simulink model "solar_powered_EV_charger"  (R2021a)
settings: Solver=VariableStepAuto  StartTime=0.0  StopTime=10.0  RelTol=1e-3
libraries: spsCurrentMeasurementLib x2, spsSeriesRLCBranchLib x2, spsVoltageMeasurementLib x2, spsDiodeLib x1, spsMosfetLib x1, spsPVArrayLib x1
settings Model: Creator=hp  LastModifiedBy=hp

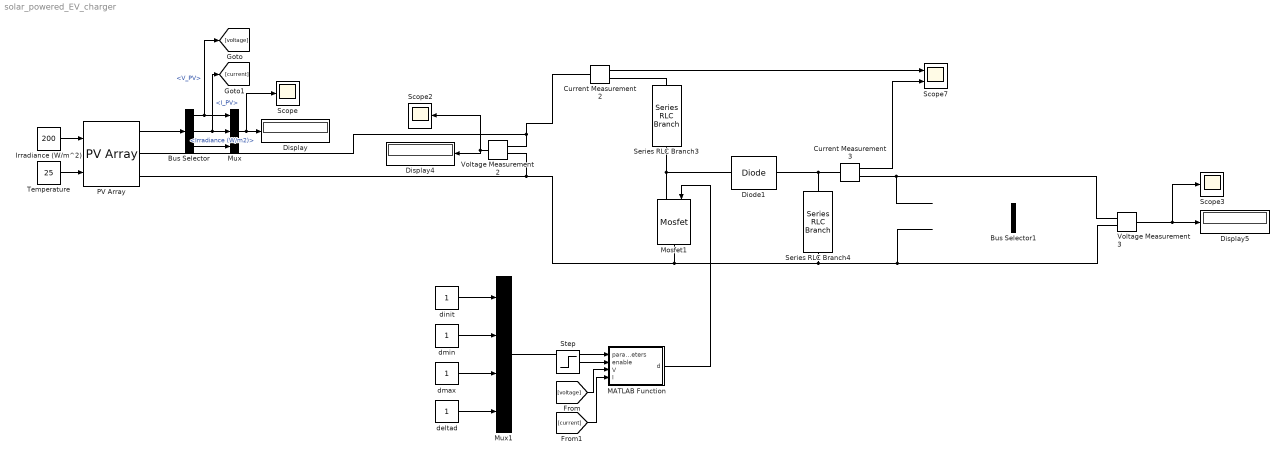
== system solar_powered_EV_charger ==
  Bus Selector : BusSelector  OutputSignals=V_PV,I_PV,Irradiance (W/m2)
  Bus Selector1 : BusSelector  OutputSignals=SOC (%),Current (A),Voltage (V)
  Current Measurement2 : spsCurrentMeasurementLib/Current Measurement  PhasorSimulation=off  OutputType=Complex  PSBequivalent=0
  Current Measurement3 : spsCurrentMeasurementLib/Current Measurement  PhasorSimulation=off  OutputType=Complex  PSBequivalent=0
  Diode1 : spsDiodeLib/Diode  Ron=0.001  Lon=0  Vf=0.8  IC=0  UseSnubber=0  Rs=500  Cs=250e-9  Measurements=off
  Display : Display
  Display4 : Display
  Display5 : Display
  Irradiance (W/m^2) : Constant  Value=200
  MATLAB Function : MATLAB Function  TreatAsAtomicUnit=on
  Mosfet1 : spsMosfetLib/Mosfet  Ron=0.1  Lon=0  Rd=0.01  Vfd=0  IC=0  Rs=1e5  Cs=inf  Measurements=off
  Mux : Mux  Inputs=3
  Mux1 : Mux
  PV Array : spsPVArrayLib/PV Array  Npar=40  Nser=10  PlotType=array @ 1000 W/m2 & specified temperatures  S_vec="[ 1000  500  100 ]"  Temp_C_vec=[45 25]  ModuleName=A10Green Technology A10J-S72-180  PlotWhenSelected=off  Pm=179.928  Ncell=72  Voc=44.06  Isc=5.31  Vm=36.72  Im=4.9  beta_Voc_pc=-0.3616  alpha_Isc_pc=0.041507  beta_Voc=-0.15932  alpha_Isc=0.002204  IL=5.3186  I0=1.8308e-10  nI=0.99015  Rsh=227.068  Rs=0.36738  RobustModel=off  RobustCellTemperature=313.3991  BAL=on  Tc=1e-6  Tfilter=5e-5
  Scope : Scope
  Scope2 : Scope
  Scope3 : Scope
  Scope7 : Scope  NumInputPorts=2
  Series RLC Branch3 : spsSeriesRLCBranchLib/Series RLC Branch  LConnTagsString=__new0  RConnTagsString=__new0  BranchType=L  Resistance=1  Inductance=1e-3  SetiL0=off  InitialCurrent=0  Capacitance=1e-6  Setx0=off  InitialVoltage=0  Measurements=None
  Series RLC Branch4 : spsSeriesRLCBranchLib/Series RLC Branch  LConnTagsString=__new0  RConnTagsString=__new0  BranchType=C  Resistance=1  Inductance=1e-3  SetiL0=off  InitialCurrent=0  Capacitance=100e-6  Setx0=off  InitialVoltage=0  Measurements=None
  Step : Step  Time=0.0001  SampleTime=0
  Temperature : Constant  Value=25
  Voltage Measurement2 : spsVoltageMeasurementLib/Voltage Measurement  PhasorSimulation=off  OutputType=Complex  PSBequivalent=0
  Voltage Measurement3 : spsVoltageMeasurementLib/Voltage Measurement  PhasorSimulation=off  OutputType=Complex  PSBequivalent=0
  deltad : Constant
  dinit : Constant
  dmax : Constant
  dmin : Constant
  wires:
  PV Array/1 -> Bus Selector/1
  Bus Selector/2 -> [current], Mux/2  "<I_PV>"
  Bus Selector/1 -> Mux/1, [voltage]  "<V_PV>"
  Bus Selector/3 -> Mux/3  "<Irradiance (W/m2)>"
  Mux/1 -> Scope/1, Display/1
  Irradiance (W/m^2)/1 -> PV Array/1
  Temperature/1 -> PV Array/2
  Current Measurement2/1 -> Scope7/1
  Current Measurement3/1 -> Scope7/2
  Voltage Measurement2/1 -> Scope2/1, Display4/1
  Voltage Measurement3/1 -> Scope3/1, Display5/1
  MATLAB Function/1(d) -> Mosfet1/1
  dinit/1 -> Mux1/1
  dmin/1 -> Mux1/2
  dmax/1 -> Mux1/3
  deltad/1 -> Mux1/4
  Mux1/1 -> MATLAB Function/1(parameters)
  Step/1 -> MATLAB Function/2(enable)
  [voltage] -> MATLAB Function/3(V)
  [current] -> MATLAB Function/4(I)
  ? -> Bus Selector1/1
  connections:
  Voltage Measurement2/LConn2 -- Voltage Measurement3/LConn2 -- Series RLC Branch4/RConn1 -- Mosfet1/RConn1 -- PV Array/RConn2
  Diode1/RConn1 -- Series RLC Branch4/LConn1 -- Current Measurement3/LConn1
  Current Measurement3/RConn1 -- Voltage Measurement3/LConn1
  Series RLC Branch3/RConn1 -- Diode1/LConn1 -- Mosfet1/LConn1
  Current Measurement2/LConn1 -- PV Array/RConn1 -- Voltage Measurement2/LConn1
  Current Measurement2/RConn1 -- Series RLC Branch3/LConn1

== matlab function solar_powered_EV_charger/MATLAB Function ==
  data: parameters input; d output; enable input; V input; I input
function d = pando(parameters,enable,V,I)
parameters(1)= Dinit;
parameters(2)= Dmin;
parameters(3)= Dmax;
parameters(4)= deltad;
data type = 'double';
persistent vold= 0, dold=dinit, pold= 0;
P=V*I;
if (P-pold~=0&&enable~=0)
    if(P-pold>0)
        if (V-Vold>0)
            d=dold-deltad;
        else
            d=dold+deltad;
        end
    else if(P-pold<0)
            if(V-vold<<0)
                d=dold-deltad;
            else
                d=dold+deltad;
            end
        end
    end
else
    d=dold;
    
            
            
           
y = u;
